simulink library "microCHP_constant"  (R2016b)
settings: Solver=ode45  StartTime=0.0  StopTime=10.0  RelTol=1e-3  EnableMultiTasking=on
undefined symbols (not defined in the file): path_carnot
libraries: carnot x4
settings Model: Creator=lena.frank  LastModifiedBy=drhf
settings DataIOCC: LimitDataPoints=on  SaveFormat=Array  SignalLoggingSaveFormat=ModelDataLogs
settings OptimizationCC: ExpressionDepthLimit=2147483647  LifeSpan=inf
settings DebuggingCC: UnderspecifiedInitializationDetection=Classic  MergeDetectMultiDrivingBlocksExec=none  SolverPrmCheckMsg=warning  FcnCallInpInsideContextMsg=warning  StateNameClashWarn=warning  SFUnexpectedBacktrackingDiag=warning  SFNoUnconditionalDefaultTransitionDiag=warning  SFExecutionAtInitializationDiag=none
settings HardwareCC: ProdBitPerPointer=32  ProdBitPerSizeT=32  ProdBitPerPtrDiffT=32  ProdLargestAtomicFloat=None  ProdIntDivRoundTo=Undefined  ProdEndianess=Unspecified  ProdWordSize=32  ProdHWDeviceType=32-bit Generic
settings ModelReferenceCC: PropagateSignalLabelsOutOfModel=off
settings GRTTargetCC: TargetLangStandard=C89/C90 (ANSI)  GeneratePreprocessorConditionals=Disable all  CombineOutputUpdateFcns=off  GRTInterface=on
settings ConfigComp: CovMetricSettings=dw  CovHtmlReporting=on  CovSaveCumulativeToWorkspaceVar=on  CovSaveSingleToWorkspaceVar=on  CovExternalEMLEnable=off

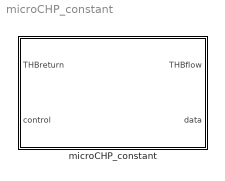
== system microCHP_constant ==
  microCHP_constant : Subsystem  mask{P_th=11520, P_el=5500, P_fuel=22030, T_flow_setpoint=80, T_return_max=75}
      mask prompts: P_th "Nominal heating power [W] - at T_flow_out of 60°C"; P_el "Electrical power [W]"; P_fuel "Fuel power [W]"; T_flow_setpoint "T_flow_setpoint [°C] - Setpoint temperature of thermostat"; T_return_max "T_return_max [°C] - safety shutdown temperature"
      mask help:
      | This block is based on characteristic curves calculating heating capacity and representing a thermostat-controlled three-way mixer valve situated in the inlet flow of a gas driven micro-CHP called "Dachs" by Senertec. External mass flow rate, outlet flow temperature and heating power factor depend on inlet return temperature and are calculated by 1-D lookup-tables based on measured data.
      | The scaling is based on a heating power of 12.52 kW, an electrical power of 5.5 kW, a fuel power of 22,03 kW and a maximum external mass flow rate of 0.14 kg/s.
      | Mass flow rate and thermal inertia are linearly resized according to the inputed nominal heating power.
      mask Help: eval('filetest (''manual.htm#electric_heating'')')
      mask Display: plot(0,0,100,100,[50,50,60,40,50],[55,40,70,60,90],[59,50],[48,40])

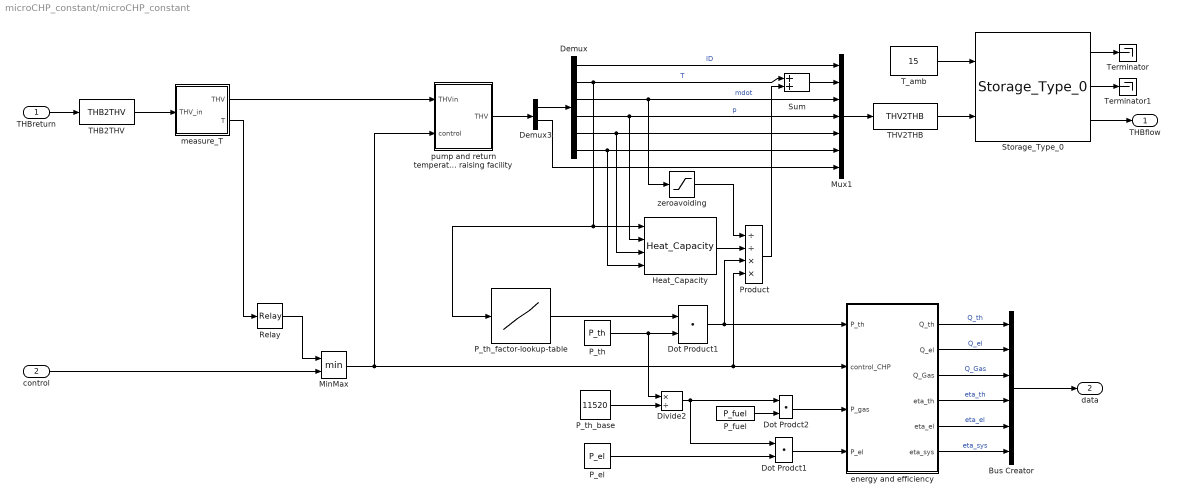
== system microCHP_constant/microCHP_constant ==
  THBreturn : Inport
  control : Inport  Port=2
  Bus Creator : BusCreator  Inputs=6
  Demux : Demux  Outputs=[1 1 1 1 1 1]
  Demux3 : Demux  Outputs=[6 14]
  Divide2 : Product  Inputs=*/
  Dot Prodct1 : DotProduct  InputSameDT=on  OutDataTypeStr=Inherit: Inherit via internal rule
  Dot Prodct2 : DotProduct  InputSameDT=on  OutDataTypeStr=Inherit: Inherit via internal rule
  Dot Product1 : DotProduct  InputSameDT=on  OutDataTypeStr=Inherit: Inherit via internal rule
  Heat_Capacity : carnot/Basic/Material_Properties/Heat_Capacity  VariantControl=CarlibClassic  INPUTARGUMENTS=state variables (classic)  DEBUGLEVEL=DEBUGLEVEL  MAXTOTALWARNINGS=inf  MAXCONSECUTIVEWARNINGS=inf  WRITETOFILE=0  FILENAME='errors.txt'
  MinMax : MinMax  Inputs=2
  Mux1 : Mux  Inputs=[1 1 1 1 1 1 14]
  P_el : Constant  Value=P_el
  P_fuel : Constant  Value=P_fuel
  P_th : Constant  Value=P_th
  P_th_base : Constant  Value=11520
  P_th_factor-lookup-table : Lookup_n-D  NumberOfTableDimensions=1  BreakpointsForDimension1=[45,50,60,65,74]  BreakpointsForDimension2=[44,80]  BreakpointsForDimension3=[1:2]  BreakpointsForDimension4=[1:2]  Table=[1.09 1.06 1 0.98 0.94]  InputSameDT=on
  Product : Product  Inputs=//**  SaturateOnIntegerOverflow=on  RndMeth=Zero  InputSameDT=on  OutDataTypeStr=Inherit: Same as first input
  Relay : Relay  OnSwitchValue=T_return_max  OffSwitchValue=T_return_max-1  OnOutputValue=0  OffOutputValue=1
  Storage_Type_0 : carnot/Storage/Thermal/Storage_Type_0  t0=25  hgt=0.63662  stgtype=0  mpts=[1 2 3 4 5 6 7 8 9 10]  tini=[25 25 25 25 25 25 25 25 25 25]  PathName=fullfile(path_carnot('libsl'),'Storage','Thermal','Storage_Type_0','parameter_set')  FileName='<user defined>'  userPath=off  userParam=on  uwall=1  ubot=1  utop=1  axcond=1  volume=0.02  dia=0.2  standing=standing cylinder  nodes=10  mpoints=10  Tsensor=0.5  pipe1inlet=1  pipe1outlet=0  pipe1dia=0.03
  Sum : Sum  SaturateOnIntegerOverflow=on  InputSameDT=on  OutDataTypeStr=Inherit: Same as first input
  THB2THV : carnot/Toolbox/THB2THV
  THV2THB : carnot/Toolbox/THV2THB
  T_amb : Constant  Value=15
  Terminator : Terminator
  Terminator1 : Terminator
  energy and efficiency : Subsystem
  measure_T : Subsystem  mask(temperature measurement sensor){tc=10, t0=25}
      mask prompts: tc "time constant of sensor [s]"; t0 "initial temperature [degree centigrade]"
      mask help: Measurement sensor for temperatures with first-oder hold. Temperature is in degree centigrade.
      mask init:
      | tc = 1/max(tc, 0.001);
      mask Help: eval('man (''measure_T'')')
      mask Display: plot(-18,0,30,20,[0 20],[0 0],[10 10 8 8 12 12 10],[0 8 8 17 17 8 8],[10 10 9 9 11 11 10 9],[15 10 10 9 9 10 9 10])
  pump and return temperature raising facility : Subsystem  mask(Pump and return temperature raising facility){fluid_id=water, mix=0, dia=0.02, power=100, p0=3e5}
      mask prompts: fluid_id "fluid"; mix "percentage of fluid mix [0..1]"; dia "diameter at in- and outlet [m]"; power "electric power consumption [W]"; p0 "system pressure [Pa]"
      mask help:
      | In this modul a pump and a return temperature raising facility are modelled by two lookup-tables. They are based on measured data.
      |
      | The mass flow-lookup table gives out the mass flow (outside of CHP) depending on the return flow temperature T_return (outside of CHP). The return flow temperature (inside of CHP) is kept on 74°C by means of a thermostatic mixing valve.
      |
      | The T_flow-lookup table gives out the flow temperature T_flow depending on the return flow temperature (outside of CHP).
      |
      | The mass flow (outside of CHP) varies by means of multiplication with a factor f_flowSetpoint depending on the flow setpoint temperature T_flowSetpoint.
      | f_flowSetpoint is calculated according to the following formula:
      | (T_flow-T_return)/(T_flowSetpoint-T_return).
      |
      | The mass flow (outside of CHP) depends also on the nominal heating power P_heating and is therefor multiplied with a factor f_power.
      | f_power is calculated according to the following formula: P_heating/11520.
      mask init:
      | mix = min(1, max(0, mix));
      | dia = max(0.001, dia);
      | p0 = max(p0, 1e5);
      mask Help: eval('htmlhelp (''chap_4_2p.htm#pump_const'')')
      mask TypeOptions fluid_id: water | air | cotton_oil | silicone_oil | water_glycol_mix
      mask Display: plot(0,0,100,100,[40,70,40,30,30,40,60,70,70,60,40],[70,50,30,40,60,70,70,60,40,30,30])
  zeroavoiding : Saturate  UpperLimit=inf  LowerLimit=1e-5
  THBflow : Outport
  data : Outport  Port=2
  wires:
  Storage_Type_0/2 -> Terminator1/1
  Relay/1 -> MinMax/1
  Bus Creator/1 -> data/1
  measure_T/1(THV) -> pump and return temperature raising facility/1(THVin)
  Dot Prodct2/1 -> energy and efficiency/3(P_gas)
  Divide2/1 -> Dot Prodct2/1, Dot Prodct1/1
  P_el/1 -> Dot Prodct1/2
  Dot Prodct1/1 -> energy and efficiency/4(P_el)
  P_fuel/1 -> Dot Prodct2/2
  P_th_base/1 -> Divide2/2
  control/1 -> MinMax/2
  MinMax/1 -> energy and efficiency/2(control_CHP), Product/4, pump and return temperature raising facility/2(control)
  Dot Product1/1 -> energy and efficiency/1(P_th), Product/3
  measure_T/2(T) -> Relay/1
  Demux/2 -> Sum/1, Heat_Capacity/1, P_th_factor-lookup-table/1  "T"
  Product/1 -> Sum/2
  pump and return temperature raising facility/1(THV) -> Demux3/1
  THBreturn/1 -> THB2THV/1
  P_th/1 -> Divide2/1, Dot Product1/2
  P_th_factor-lookup-table/1 -> Dot Product1/1
  Mux1/1 -> THV2THB/1
  Demux3/2 -> Mux1/7
  Demux3/1 -> Demux/1
  Sum/1 -> Mux1/2
  zeroavoiding/1 -> Product/1
  Demux/3 -> zeroavoiding/1, Mux1/3  "mdot"
  Heat_Capacity/1 -> Product/2
  Demux/6 -> Mux1/6, Heat_Capacity/4
  Demux/5 -> Mux1/5, Heat_Capacity/3
  Demux/1 -> Mux1/1  "ID"
  Demux/4 -> Mux1/4, Heat_Capacity/2  "p"
  THV2THB/1 -> Storage_Type_0/2
  THB2THV/1 -> measure_T/1(THV_in)
  Storage_Type_0/3 -> THBflow/1
  Storage_Type_0/1 -> Terminator/1
  T_amb/1 -> Storage_Type_0/1
  energy and efficiency/6(eta_sys) -> Bus Creator/6  "eta_sys"
  energy and efficiency/5(eta_el) -> Bus Creator/5  "eta_el"
  energy and efficiency/4(eta_th) -> Bus Creator/4  "eta_th"
  energy and efficiency/3(Q_Gas) -> Bus Creator/3  "Q_Gas"
  energy and efficiency/2(Q_el) -> Bus Creator/2  "Q_el"
  energy and efficiency/1(Q_th) -> Bus Creator/1  "Q_th"

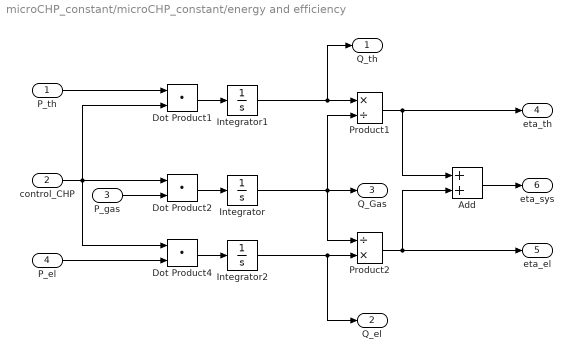
== system microCHP_constant/microCHP_constant/energy and efficiency ==
  P_th : Inport
  control_CHP : Inport  Port=2
  P_gas : Inport  Port=3
  P_el : Inport  Port=4
  Add : Sum
  Dot Product1 : DotProduct  InputSameDT=on  OutDataTypeStr=Inherit: Inherit via internal rule
  Dot Product2 : DotProduct  InputSameDT=on  OutDataTypeStr=Inherit: Inherit via internal rule
  Dot Product4 : DotProduct  InputSameDT=on  OutDataTypeStr=Inherit: Inherit via internal rule
  Integrator : Integrator
  Integrator1 : Integrator
  Integrator2 : Integrator
  Product1 : Product  Inputs=*/  SaturateOnIntegerOverflow=on  RndMeth=Zero  InputSameDT=on  OutDataTypeStr=Inherit: Same as first input
  Product2 : Product  Inputs=/*  SaturateOnIntegerOverflow=on  RndMeth=Zero  InputSameDT=on  OutDataTypeStr=Inherit: Same as first input
  Q_th : Outport
  Q_el : Outport  Port=2
  Q_Gas : Outport  Port=3
  eta_th : Outport  Port=4
  eta_el : Outport  Port=5
  eta_sys : Outport  Port=6
  wires:
  Add/1 -> eta_sys/1
  Product1/1 -> eta_th/1, Add/1
  Integrator1/1 -> Q_th/1, Product1/1
  P_th/1 -> Dot Product1/1
  Dot Product1/1 -> Integrator1/1
  Integrator2/1 -> Q_el/1, Product2/2
  Integrator/1 -> Product1/2, Q_Gas/1, Product2/1
  control_CHP/1 -> Dot Product1/2, Dot Product4/1, Dot Product2/1
  Dot Product2/1 -> Integrator/1
  Dot Product4/1 -> Integrator2/1
  Product2/1 -> Add/2, eta_el/1
  P_el/1 -> Dot Product4/2
  P_gas/1 -> Dot Product2/2

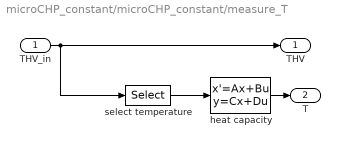
== system microCHP_constant/microCHP_constant/measure_T ==
  THV_in : Inport
  heat capacity : StateSpace  A=-tc  B=tc  D=0  X0=t0
  select temperature : Selector  InputPortWidth=20  IndexOptions=Index vector (dialog)  Indices=[2]  OutputSizes=1
  THV : Outport
  T : Outport  Port=2
  wires:
  heat capacity/1 -> T/1
  select temperature/1 -> heat capacity/1
  THV_in/1 -> THV/1, select temperature/1

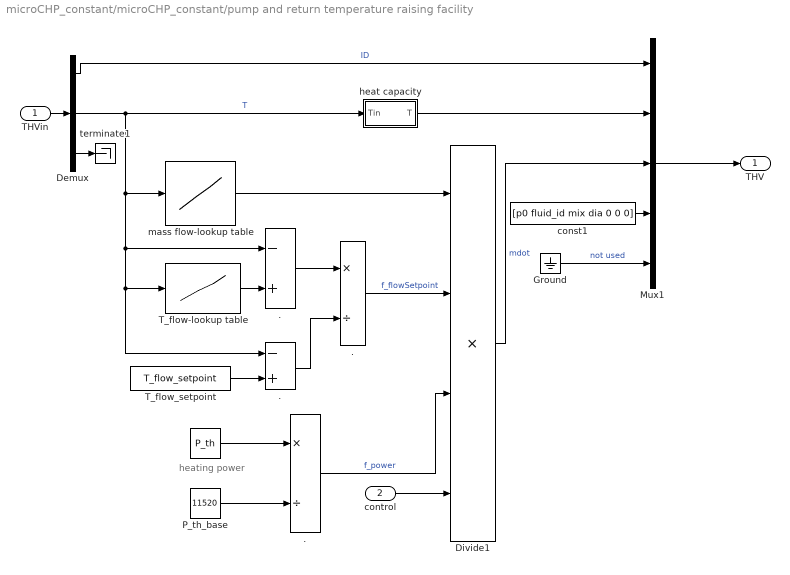
== system microCHP_constant/microCHP_constant/pump and return temperature raising facility ==
  note: heating power
  THVin : Inport
  control : Inport  Port=2
  " " : Constant  Value=P_th
  " ." : Product  Inputs=*/
  " .  " : Sum  Inputs=-+
  . : Sum  Inputs=-+
  ". " : Product  Inputs=*/
  Demux : Demux  Outputs=[1 1 18]
  Divide1 : Product  Inputs=****
  Ground : Ground
  Mux1 : Mux  Inputs=[1 1 1 7 10]
  P_th_base : Constant  Value=11520
  T_flow-lookup table : Lookup_n-D  NumberOfTableDimensions=1  BreakpointsForDimension1=[45,50,60,65,74]  BreakpointsForDimension2=[44,80]  BreakpointsForDimension3=[1:2]  BreakpointsForDimension4=[1:2]  Table=[78.5 79.65 81 84.18 92.47]  InputSameDT=on
  T_flow_setpoint : Constant  Value=T_flow_setpoint
  const1 : Constant  Value=[p0 fluid_id mix dia 0 0 0]
  heat capacity : Subsystem  mask{NTU=3.3}
      mask prompts: NTU "NTU (k*A/(m*cp))"
  mass flow-lookup table : Lookup_n-D  NumberOfTableDimensions=1  BreakpointsForDimension1=[45,50,60,65,74]  BreakpointsForDimension2=[44,80]  BreakpointsForDimension3=[1:2]  BreakpointsForDimension4=[1:2]  Table=[0.09 0.1 0.129 0.139 0.140]  InputSameDT=on
  terminate1 : Terminator
  THV : Outport
  wires:
  control/1 -> Divide1/4
  " ."/1 -> Divide1/3  "f_power"
  ". "/1 -> Divide1/2  "f_flowSetpoint"
  P_th_base/1 -> " ."/2
  T_flow-lookup table/1 -> ./2
  T_flow_setpoint/1 -> " .  "/2
  " .  "/1 -> ". "/2
  ./1 -> ". "/1
  Divide1/1 -> Mux1/3  "mdot"
  mass flow-lookup table/1 -> Divide1/1
  " "/1 -> " ."/1
  THVin/1 -> Demux/1
  const1/1 -> Mux1/4
  Demux/3 -> terminate1/1
  heat capacity/1(T) -> Mux1/2
  Demux/2 -> " .  "/1, T_flow-lookup table/1, ./1, mass flow-lookup table/1, heat capacity/1(Tin)  "T"
  Mux1/1 -> THV/1
  Demux/1 -> Mux1/1  "ID"
  Ground/1 -> Mux1/5  "not used"

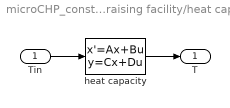
== system microCHP_constant/microCHP_constant/pump and return temperature raising facility/heat capacity ==
  Tin : Inport
  heat capacity : StateSpace  A=-NTU  B=NTU  D=0  X0=80
  T : Outport
  wires:
  Tin/1 -> heat capacity/1
  heat capacity/1 -> T/1
